simulink model "sampleModel1558"  (R2023a)
settings: Solver=VariableStepAuto  StartTime=0.0  StopTime=10.0  RelTol=1e-3
libraries: simulink x2, hdlsllib x1
settings Model: Creator=user1  LastModifiedBy=user1

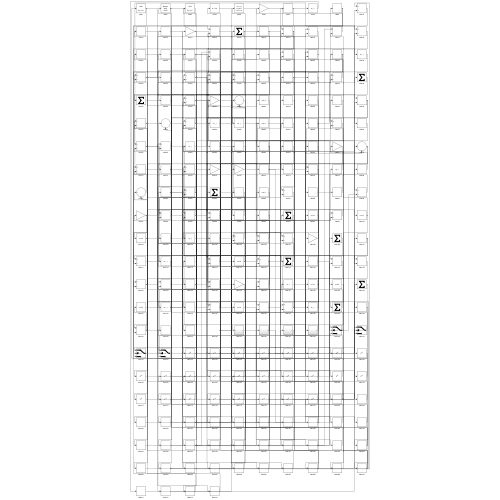
[thumbnail: Simulink's stored preview of the top-level diagram]
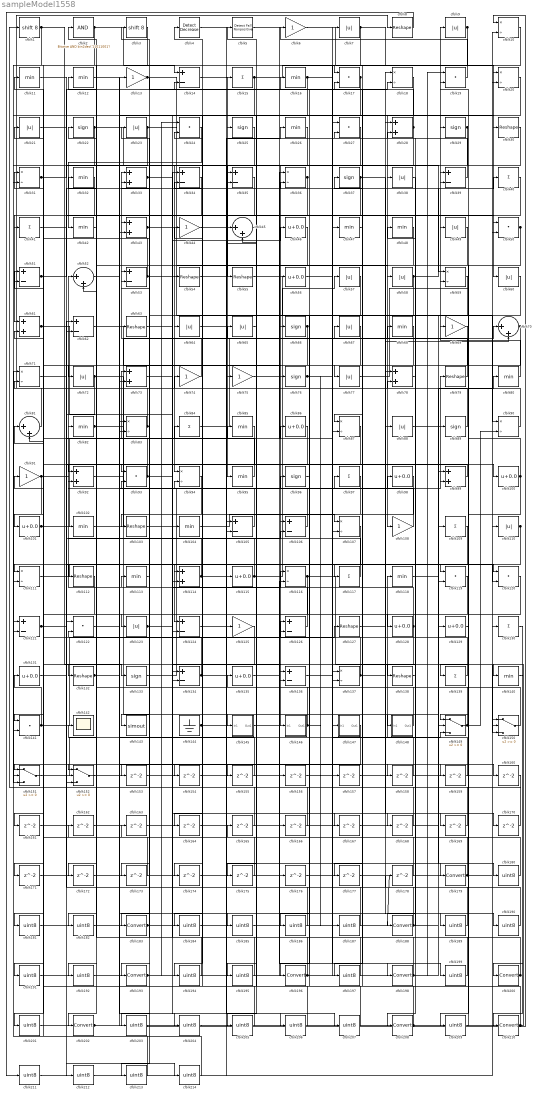
== system sampleModel1558 ==
  cfblk1 : ArithShift  BitShiftNumber=8
  cfblk{10,18,20,31,36,59,71,83,87,90,94,107,111,116,137} (15 alike) : Product  Inputs=*/  RndMeth=Zero  SaturateOnIntegerOverflow=on
  cfblk{46,56,86,98,100..101,115,128..129,131,135} (11 alike) : Bias  Bias=0.0  SaturateOnIntegerOverflow=off
  cfblk{11..12,16,26,32,42,47..48,68,80,82,85,95,102,104,113,118,140} (18 alike) : MinMax
  cfblk{8,30,54..55,63,79,103,112,127,132,138} (11 alike) : Reshape
  cfblk{14,34..35,39,51,53,62,105..106,121,124,126,134,136} (14 alike) : Sum  Inputs=+-
  cfblk{6,13,44,69,74..75,91,108,125} (9 alike) : Gain
  cfblk{15,40..41,84,97,109,117,130,139} (9 alike) : Sum  Inputs=+
  cfblk{7,9,21,23,38,49,57..58,60,64..65,67,72,77,88,110,123} (17 alike) : Abs  SaturateOnIntegerOverflow=off
  cfblk{28,33,43,61,73,78,92,99,114} (9 alike) : Sum
  cfblk{17,19,24,27,50,93,119..120,122,141} (10 alike) : DotProduct  OutDataTypeStr=Inherit: Inherit via internal rule
  cfblk{22,25,29,37,66,76,89,96,133} (9 alike) : Signum
  cfblk142 : Scope
  cfblk143 : ToWorkspace  VariableName=simout  SaveFormat=Timeseries  SampleTime=-1
  cfblk144 : Ground
  cfblk145 : Subsystem
      settings: LibrarySourceBlock=|
      | hdlsllib/Ports &
      | Subsystems/Subsystem
  cfblk146 : Subsystem
      settings: LibrarySourceBlock=|
      | hdlsllib/Ports &
      | Subsystems/Subsystem
  cfblk147 : Subsystem
      settings: LibrarySourceBlock=|
      | hdlsllib/Ports &
      | Subsystems/Subsystem
  cfblk148 : Subsystem
      settings: LibrarySourceBlock=|
      | hdlsllib/Ports &
      | Subsystems/Subsystem
  cfblk{149..152} (4 alike) : Switch  SaturateOnIntegerOverflow=off  InputSameDT=off
  cfblk{153..178} (26 alike) : Delay  SampleTime=1
  cfblk{179,183,188,193,196,198,200,202,208,210} (10 alike) : DataTypeConversion  SaturateOnIntegerOverflow=off  RndMeth=Floor
  cfblk{180..182,184..187,189..192,194..195,197,199,201,203..207,209,211..214} (26 alike) : DataTypeConversion  OutDataTypeStr=uint8  SaturateOnIntegerOverflow=off  RndMeth=Floor
  cfblk2 : simulink/Logic and Bit Operations/Bitwise Operator  logicop=AND  UseBitMask=on  BitMask=bin2dec('11011001')  BitMaskRealWorld=Stored Integer
      settings: LibrarySourceBlock=|
      | hdlsllib/Logic and Bit
      | Operations/Bitwise
      | Operator
  cfblk3 : ArithShift  BitShiftNumber=8
  cfblk4 : simulink/Logic and Bit Operations/Detect Decrease  vinit=0.0  OutDataTypeStr=boolean
      settings: LibrarySourceBlock=|
      | hdlsllib/Logic and Bit
      | Operations/Detect
      | Decrease
  cfblk{45,52,70,81} (4 alike) : Sum  Inputs=|++
  cfblk5 : hdlsllib/Logic and Bit Operations/Detect Fall Nonpositive  vinit=0  OutDataTypeStr=boolean
  wires:
  cfblk39/1 -> cfblk15/1
  cfblk58/1 -> cfblk40/1, cfblk186/1
  cfblk151/1 -> cfblk118/1
  cfblk50/1 -> cfblk139/1, cfblk112/1
  cfblk26/1 -> cfblk94/1
  cfblk54/1 -> cfblk25/1
  cfblk38/1 -> cfblk67/1
  cfblk82/1 -> cfblk145/1(In1), cfblk204/1
  cfblk1/1 -> cfblk133/1, cfblk151/3
  cfblk24/1 -> cfblk42/1
  cfblk137/1 -> cfblk12/1, cfblk70/2
  cfblk18/1 -> cfblk108/1
  cfblk30/1 -> cfblk95/1
  cfblk136/1 -> cfblk27/1
  cfblk119/1 -> cfblk128/1
  cfblk133/1 -> cfblk79/1
  cfblk139/1 -> cfblk22/1
  cfblk15/1 -> cfblk17/1, cfblk114/2
  cfblk84/1 -> cfblk70/1
  cfblk13/1 -> cfblk58/1, cfblk103/1
  cfblk10/1 -> cfblk202/1
  cfblk77/1 -> cfblk9/1
  cfblk80/1 -> cfblk49/1
  cfblk6/1 -> cfblk60/1
  cfblk130/1 -> cfblk210/1
  cfblk79/1 -> cfblk33/1
  cfblk81/1 -> cfblk8/1
  cfblk57/1 -> cfblk143/1
  cfblk132/1 -> cfblk99/2, cfblk126/1
  cfblk128/1 -> cfblk52/1, cfblk141/1
  cfblk21/1 -> cfblk50/1
  cfblk19/1 -> cfblk6/1
  cfblk22/1 -> cfblk115/1, cfblk121/2
  cfblk114/1 -> cfblk82/1, cfblk149/2
  cfblk100/1 -> cfblk29/1, cfblk149/1
  cfblk148/1(Out1) -> cfblk113/1
  cfblk28/1 -> cfblk3/1, cfblk153/1
  cfblk34/1 -> cfblk193/1
  cfblk108/1 -> cfblk32/1
  cfblk110/1 -> cfblk120/2, cfblk172/1
  cfblk37/1 -> cfblk160/1, cfblk161/1
  cfblk9/1 -> cfblk87/2, cfblk177/1
  cfblk135/1 -> cfblk198/1
  cfblk36/1 -> cfblk52/2, cfblk92/1
  cfblk17/1 -> cfblk55/1, cfblk111/2
  cfblk138/1 -> cfblk48/1
  cfblk92/1 -> cfblk124/1
  cfblk149/1 -> cfblk23/1, cfblk90/2
  cfblk41/1 -> cfblk119/1
  cfblk115/1 -> cfblk57/1, cfblk92/2
  cfblk61/1 -> cfblk134/1, cfblk214/1
  cfblk27/1 -> cfblk146/1(In1)
  cfblk14/1 -> cfblk66/1
  cfblk48/1 -> cfblk64/1
  cfblk62/1 -> cfblk76/1
  cfblk11/1 -> cfblk100/1
  cfblk104/1 -> cfblk107/1
  cfblk87/1 -> cfblk101/1
  cfblk112/1 -> cfblk151/1
  cfblk55/1 -> cfblk129/1
  cfblk68/1 -> cfblk77/1
  cfblk66/1 -> cfblk124/2, cfblk111/1
  cfblk117/1 -> cfblk84/1
  cfblk72/1 -> cfblk137/2, cfblk152/3
  cfblk74/1 -> cfblk63/1
  cfblk56/1 -> cfblk148/1(In1)
  cfblk90/1 -> cfblk19/2
  cfblk12/1 -> cfblk30/1
  cfblk101/1 -> cfblk36/1, cfblk201/1
  cfblk43/1 -> cfblk88/1, cfblk120/1
  cfblk23/1 -> cfblk59/1, cfblk141/2, cfblk170/1
  cfblk69/1 -> cfblk208/1
  cfblk102/1 -> cfblk56/1
  cfblk152/1 -> cfblk47/1
  cfblk146/1(Out1) -> cfblk102/1, cfblk157/1
  cfblk144/1 -> cfblk26/1, cfblk149/3
  cfblk98/1 -> cfblk106/1
  cfblk4/1 -> cfblk179/1
  cfblk32/1 -> cfblk61/1
  cfblk7/1 -> cfblk20/1, cfblk41/1
  cfblk78/1 -> cfblk188/1
  cfblk29/1 -> cfblk54/1, cfblk175/1
  cfblk93/1 -> cfblk31/1, cfblk68/1
  cfblk51/1 -> cfblk36/2, cfblk81/2
  cfblk53/1 -> cfblk21/1, cfblk90/1
  cfblk33/1 -> cfblk39/2, cfblk206/1
  cfblk2/1 -> cfblk14/1, cfblk31/2
  cfblk49/1 -> cfblk138/1
  cfblk46/1 -> cfblk72/1
  cfblk123/1 -> cfblk116/1, cfblk43/1
  cfblk91/1 -> cfblk7/1, cfblk151/2
  cfblk125/1 -> cfblk183/1
  cfblk5/1 -> cfblk107/2
  cfblk121/1 -> cfblk51/1, cfblk85/1
  cfblk86/1 -> cfblk152/1
  cfblk95/1 -> cfblk73/1
  cfblk116/1 -> cfblk150/3, cfblk195/1
  cfblk126/1 -> cfblk14/2
  cfblk141/1 -> cfblk127/1, cfblk131/1
  cfblk83/1 -> cfblk123/1, cfblk2/1
  cfblk105/1 -> cfblk74/1
  cfblk31/1 -> cfblk38/1, cfblk18/2
  cfblk16/1 -> cfblk114/1, cfblk199/1
  cfblk150/1 -> cfblk44/1
  cfblk88/1 -> cfblk80/1
  cfblk111/1 -> cfblk117/1
  cfblk63/1 -> cfblk46/1
  cfblk120/1 -> cfblk152/2
  cfblk59/1 -> cfblk87/1
  cfblk76/1 -> cfblk39/1, cfblk187/1
  cfblk40/1 -> cfblk62/2
  cfblk103/1 -> cfblk86/1
  cfblk113/1 -> cfblk53/1
  cfblk70/1 -> cfblk173/1, cfblk174/1
  cfblk106/1 -> cfblk65/1
  cfblk134/1 -> cfblk98/1, cfblk24/2, cfblk11/1
  cfblk89/1 -> cfblk51/2
  cfblk96/1 -> cfblk196/1
  cfblk3/1 -> cfblk132/1
  cfblk140/1 -> cfblk200/1
  cfblk131/1 -> cfblk106/2
  cfblk99/1 -> cfblk93/1
  cfblk20/1 -> cfblk83/2
  cfblk73/1 -> cfblk136/1
  cfblk153/1 -> cfblk150/1
  cfblk67/1 -> cfblk154/1
  cfblk65/1 -> cfblk155/1
  cfblk155/1 -> cfblk83/1
  cfblk156/1 -> cfblk28/1
  cfblk157/1 -> cfblk150/2
  cfblk124/1 -> cfblk158/1
  cfblk158/1 -> cfblk17/2
  cfblk52/1 -> cfblk159/1
  cfblk159/1 -> cfblk137/1
  cfblk160/1 -> cfblk1/1
  cfblk161/1 -> cfblk136/2
  cfblk162/1 -> cfblk134/2
  cfblk163/1 -> cfblk93/2
  cfblk60/1 -> cfblk164/1
  cfblk164/1 -> cfblk99/1
  cfblk165/1 -> cfblk53/2
  cfblk145/1(Out1) -> cfblk166/1
  cfblk166/1 -> cfblk121/1
  cfblk75/1 -> cfblk167/1
  cfblk167/1 -> cfblk18/1
  cfblk64/1 -> cfblk168/1
  cfblk168/1 -> cfblk62/1
  cfblk127/1 -> cfblk169/1
  cfblk169/1 -> cfblk81/1
  cfblk170/1 -> cfblk105/1
  cfblk35/1 -> cfblk171/1
  cfblk171/1 -> cfblk73/2
  cfblk172/1 -> cfblk50/2
  cfblk173/1 -> cfblk61/2
  cfblk174/1 -> cfblk116/2
  cfblk175/1 -> cfblk33/2
  cfblk176/1 -> cfblk20/2
  cfblk178/1 -> cfblk97/1
  cfblk179/1 -> cfblk110/1, cfblk5/1, cfblk35/1
  cfblk118/1 -> cfblk180/1
  cfblk180/1 -> cfblk4/1
  cfblk109/1 -> cfblk181/1
  cfblk181/1 -> cfblk104/1
  cfblk85/1 -> cfblk182/1
  cfblk182/1 -> cfblk109/1
  cfblk183/1 -> cfblk178/1, cfblk35/2
  cfblk97/1 -> cfblk184/1
  cfblk184/1 -> cfblk125/1
  cfblk122/1 -> cfblk185/1
  cfblk185/1 -> cfblk156/1
  cfblk186/1 -> cfblk122/1
  cfblk187/1 -> cfblk122/2
  cfblk188/1 -> cfblk126/2, cfblk28/2
  cfblk177/1 -> cfblk189/1
  cfblk189/1 -> cfblk78/1
  cfblk44/1 -> cfblk190/1
  cfblk190/1 -> cfblk78/2
  cfblk147/1(Out1) -> cfblk191/1
  cfblk191/1 -> cfblk13/1
  cfblk42/1 -> cfblk192/1
  cfblk192/1 -> cfblk147/1(In1)
  cfblk193/1 -> cfblk176/1, cfblk24/1, cfblk89/1
  cfblk25/1 -> cfblk194/1
  cfblk194/1 -> cfblk34/1
  cfblk195/1 -> cfblk34/2
  cfblk196/1 -> cfblk119/2, cfblk142/1
  cfblk47/1 -> cfblk197/1
  cfblk197/1 -> cfblk96/1
  cfblk198/1 -> cfblk165/1, cfblk19/1
  cfblk199/1 -> cfblk135/1
  cfblk200/1 -> cfblk163/1, cfblk162/1
  cfblk201/1 -> cfblk140/1
  cfblk202/1 -> cfblk43/2, cfblk75/1
  cfblk107/1 -> cfblk203/1
  cfblk203/1 -> cfblk10/1
  cfblk204/1 -> cfblk10/2
  cfblk45/1 -> cfblk205/1
  cfblk205/1 -> cfblk91/1
  cfblk206/1 -> cfblk45/1
  cfblk154/1 -> cfblk207/1
  cfblk207/1 -> cfblk45/2
  cfblk208/1 -> cfblk27/2, cfblk94/2
  cfblk129/1 -> cfblk209/1
  cfblk209/1 -> cfblk69/1
  cfblk210/1 -> cfblk16/1, cfblk59/2, cfblk37/1
  cfblk8/1 -> cfblk211/1
  cfblk211/1 -> cfblk130/1
  cfblk71/1 -> cfblk212/1
  cfblk212/1 -> cfblk105/2
  cfblk94/1 -> cfblk213/1
  cfblk213/1 -> cfblk71/1
  cfblk214/1 -> cfblk71/2

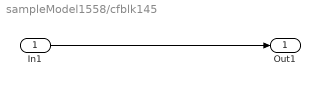
== system sampleModel1558/cfblk145 ==
  In1 : Inport
  Out1 : Outport
  wires:
  In1/1 -> Out1/1

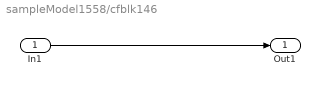
== system sampleModel1558/cfblk146 ==
  In1 : Inport
  Out1 : Outport
  wires:
  In1/1 -> Out1/1

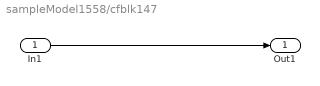
== system sampleModel1558/cfblk147 ==
  In1 : Inport
  Out1 : Outport
  wires:
  In1/1 -> Out1/1

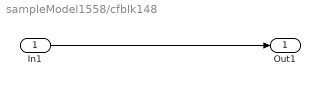
== system sampleModel1558/cfblk148 ==
  In1 : Inport
  Out1 : Outport
  wires:
  In1/1 -> Out1/1
